simulink model "FOC_simulink"  (R2020a)
settings: Solver=FixedStepAuto  StartTime=0.0  StopTime=10.0  FixedStep=PWM_Ts  RelTol=1e-3
values from neighbouring files (symbols this model uses):
  P = 2    [Motor_Parameters.m]
  PWM_Ts = 1/10000    (= 0.0001)    [Motor_Parameters.m]
  Voltage = 24    [Motor_Parameters.m]
undefined symbols (not defined in the file or in its folder): sigbuilder_block
libraries: mcbplantlib x1, autolibpmsmexterior x1
settings Model: Creator=HP  LastModifiedBy=HP

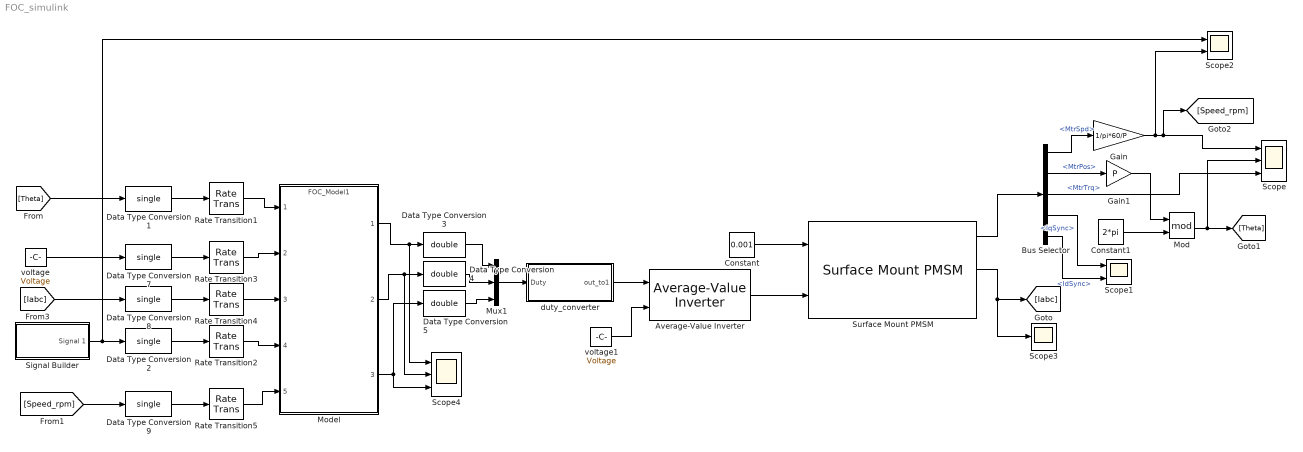
== system FOC_simulink ==
  Average-Value Inverter : mcbplantlib/Average-Value Inverter
  Bus Selector : BusSelector  OutputSignals=MtrSpd,MtrPos,MtrTrq,IqSync,IdSync
  Constant : Constant  Value=0.001
  Constant1 : Constant  Value=2*pi
  Data Type Conversion{1..2,7..9} (5 alike) : DataTypeConversion  OutDataTypeStr=single
  Data Type Conversion3 : DataTypeConversion  OutDataTypeStr=double
  Data Type Conversion4 : DataTypeConversion  OutDataTypeStr=double
  Data Type Conversion5 : DataTypeConversion  OutDataTypeStr=double
  Gain : Gain  Gain=1/pi*60/P
  Gain1 : Gain  Gain=P
  Mod : Math  Operator=mod  SaturateOnIntegerOverflow=on
  Model : ModelReference  ModelNameDialog=FOC_Model1.slx  SimulationMode=Normal  ModelReferenceVersion=1.76
  Mux1 : Mux  Inputs=3
  Rate Transition{1..5} (5 alike) : RateTransition
  Scope : Scope  NumInputPorts=3
  Scope1 : Scope  NumInputPorts=2
  Scope2 : Scope  NumInputPorts=2
  Scope3 : Scope
  Scope4 : Scope  NumInputPorts=3
  Signal Builder : Subsystem  Tag=STV Subsys  LoadFcn=sigbuilder_block('load');  StartFcn=sigbuilder_block('start');  StopFcn=sigbuilder_block('stop');  ClipboardFcn=sigbuilder_block('clipboard');  mask(Sigbuilder block){tuvar=[0:10]}
      mask help: Simulink:masks:SigbuilderBlock_MD
      mask init:
      | if ~strcmp(get_param(bdroot(gcbh),'SimulationStatus'),'stopped') tuvar = sigbuilder_block('maskInit'); end
      settings: CopyFcn=sigbuilder_block('copy');  DeleteFcn=sigbuilder_block('delete');  ModelCloseFcn=sigbuilder_block('modelClose');  PreSaveFcn=sigbuilder_block('preSave');  PauseFcn=sigbuilder_block('pause');  ContinueFcn=sigbuilder_block('continue');  NameChangeFcn=sigbuilder_block('namechange');  OpenFcn=sigbuilder_block('open',[437.6 199.2 550.4 400 ]);  CloseFcn=sigbuilder_block('close');
      mask Display: plot(0, 0, 100, 100,[2, 2, 32, 32, 2], [68, 8, 8, 68, 68],[32, 2], [38, 38], [32, 19, 2],[53, 60, 44], [32, 17, 17, 2],[16, 16, 31, 31]);txt = getActiveGroup(gcbh);text(2, 100, txt,'verticalAlignment', 'top');
  Surface Mount PMSM : autolibpmsmexterior/Surface Mount PMSM  port_config=Torque  sim_type=Discrete  Ts=PWM_Ts  P=P  Rs=Rs  Ldq_=Ls  KConstText=Permanent flux linkage constant (lambda_pm):  lambda_pm=Flux  Ke=159.9771  Kt=1.323  mechanical=[0.0001, 4.924e-4, 0]  idq0=[0 0]  theta_init=0  omega_init=0  KConst=Flux  lambda_pm_calc=Flux  RefBlkName='autolibpmsmexterior/Surface Mount PMSM'  aMode=1  Ldq="[0.0003752   0.0003752]"
      settings: SourceProductBaseCode=PW,MT,VE,VP
  duty_converter : Subsystem
  voltage : Constant  Value=Voltage
  voltage1 : Constant  Value=Voltage
  wires:
  Constant/1 -> Surface Mount PMSM/1
  Average-Value Inverter/1 -> Surface Mount PMSM/2
  duty_converter/1(out_to1) -> Average-Value Inverter/1
  Surface Mount PMSM/1 -> Bus Selector/1
  Bus Selector/1 -> Gain/1  "<MtrSpd>"
  Bus Selector/2 -> Gain1/1  "<MtrPos>"
  Bus Selector/3 -> Scope/3  "<MtrTrq>"
  Gain/1 -> Scope2/2, [Speed_rpm], Scope/1
  Gain1/1 -> Mod/1
  Mod/1 -> [Theta], Scope/2
  Constant1/1 -> Mod/2
  Surface Mount PMSM/2 -> [Iabc], Scope3/1
  Mux1/1 -> duty_converter/1(Duty)
  voltage1/1 -> Average-Value Inverter/2
  [Theta] -> Data Type Conversion1/1
  Data Type Conversion2/1 -> Rate Transition2/1
  Signal Builder/1(Signal 1) -> Scope2/1, Data Type Conversion2/1
  Model/1 -> Scope4/1, Data Type Conversion3/1
  Data Type Conversion1/1 -> Rate Transition1/1
  Rate Transition1/1 -> Model/1
  Model/2 -> Scope4/2, Data Type Conversion4/1
  Model/3 -> Scope4/3, Data Type Conversion5/1
  Data Type Conversion3/1 -> Mux1/1
  Data Type Conversion4/1 -> Mux1/2
  Data Type Conversion5/1 -> Mux1/3
  voltage/1 -> Data Type Conversion7/1
  Data Type Conversion7/1 -> Rate Transition3/1
  Rate Transition3/1 -> Model/2
  Rate Transition2/1 -> Model/4
  Data Type Conversion8/1 -> Rate Transition4/1
  [Iabc] -> Data Type Conversion8/1
  Rate Transition4/1 -> Model/3
  Bus Selector/4 -> Scope1/1  "<IqSync>"
  Bus Selector/5 -> Scope1/2  "<IdSync>"
  Data Type Conversion9/1 -> Rate Transition5/1
  [Speed_rpm] -> Data Type Conversion9/1
  Rate Transition5/1 -> Model/5

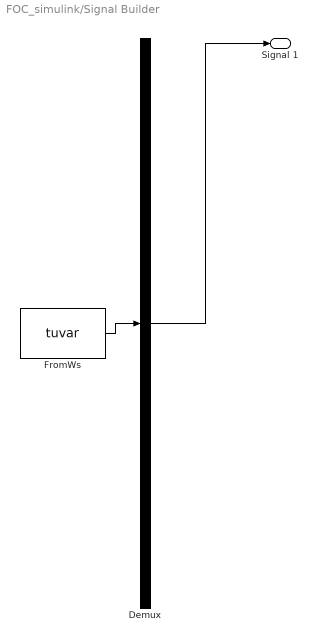
== system FOC_simulink/Signal Builder ==
  Demux : Demux  Tag=STV Demux  Outputs=1
      settings: DisplayOption=none
  FromWs : FromWorkspace  Tag=STV FromWs  VariableName=tuvar
      SigBuilderData=|
      | common.afterFinalStr = 'Extrapolate'
      | common.sampleTime = 0
      | dataSet.timeRange = [0 10]
      | dataSet.name = 'Group 1'
      | sbobj.Groups.Name = 'Group 1'
      | sbobj.Groups.Signals.Name = 'Signal 1'
      | sbobj.Groups.Signals.XData = [0 4 6 10]
      | sbobj.Groups.Signals.YData = [1000 1000 1000 1000]
  Signal 1 : Outport  Tag=STV Outport
  wires:
  Demux/1 -> Signal 1/1
  FromWs/1 -> Demux/1

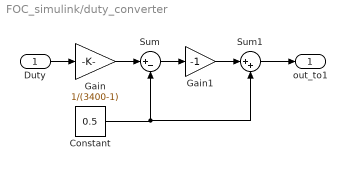
== system FOC_simulink/duty_converter ==
  Duty : Inport
  Constant : Constant  Value=0.5
  Gain : Gain  Gain=1/(3400-1)
  Gain1 : Gain  Gain=-1
  Sum : Sum  Inputs=|+-
  Sum1 : Sum  Inputs=|++
  out_to1 : Outport
  wires:
  Duty/1 -> Gain/1
  Gain/1 -> Sum/1
  Constant/1 -> Sum1/2, Sum/2
  Sum/1 -> Gain1/1
  Gain1/1 -> Sum1/1
  Sum1/1 -> out_to1/1
